simulink model "SID"  (R2017b)
settings: Solver=FixedStepAuto  StartTime=0.0  StopTime=inf  RelTol=1e-3  EnableMultiTasking=on
values from neighbouring files (symbols this model uses):
  Ad = Ad+Anew^i*Ts^i/factorial(i)    [SiD_Skript.m]
  Bd = pinv(Anew)*(Ad-eye(13))*Bnew    [SiD_Skript.m]
  Cd = C    [SiD_Skript.m]
  Dd = 0    [SiD_Skript.m]
  l = 0.175    [SiD_Skript.m]
libraries: WebSocketLibrary x1
settings Model: SimulationMode=external  Creator=seel  LastModifiedBy=jan
settings OptimizationCC: DefaultParameterBehavior=Inlined
settings DebuggingCC: MultiTaskCondExecSysMsg=warning  ParameterTunabilityLossMsg=error
settings SFSimCC: MATLABDynamicMemAlloc=off
settings RTWCC: SystemTargetFile=ert_linux.tlc  MakeCommand=make_rtw OPTS=-DWITH_HW  TemplateMakefile=ert_linux.tmf  Description=Linux Embedded Coder  GenerateReport=on  IncludeHyperlinkInReport=on  LaunchReport=on  TargetLang=C++  GenerateTraceInfo=on  GenerateTraceReport=on  GenerateTraceReportSl=on  GenerateTraceReportSf=on  GenerateTraceReportEml=on
settings CodeAppCC: ForceParamTrailComments=on  IgnoreCustomStorageClasses=off  OperatorAnnotations=on  SimulinkDataObjDesc=on  SFDataObjDesc=on  MATLABFcnDesc=on  InsertBlockDesc=on  StateflowObjectComments=on  MATLABSourceComments=on
settings STFCustomTargetCC: TargetLangStandard=C++03 (ISO)  ModelReferenceCompliant=off  CombineOutputUpdateFcns=on  ERTCustomFileBanners=on  SupportNonInlinedSFcns=off  RemoveResetFunc=on  SupportVariableSizeSignals=on  MATLABClassNameForMDSCustomization=Simulink.SoftwareTarget.ERTCustomization  GRTInterface=off  SystemTargetFile=ert_linux.tlc
settings ERTTargetCC: TargetLangStandard=C++03 (ISO)  MultiwordLength=2048  ModelReferenceCompliant=off  ParMdlRefBuildCompliant=off  CompOptLevelCompliant=off  ConcurrentExecutionCompliant=off  SupportContinuousTime=on  SupportVariableSizeSignals=on  ModelStepFunctionPrototypeControlCompliant=off  CPPClassGenCompliant=off  UseToolchainInfoCompliant=off  ExtMode=on  InlinedParameterPlacement=NonHierarchical  ERTCustomFileTemplate=ert_linux_file_process.tlc

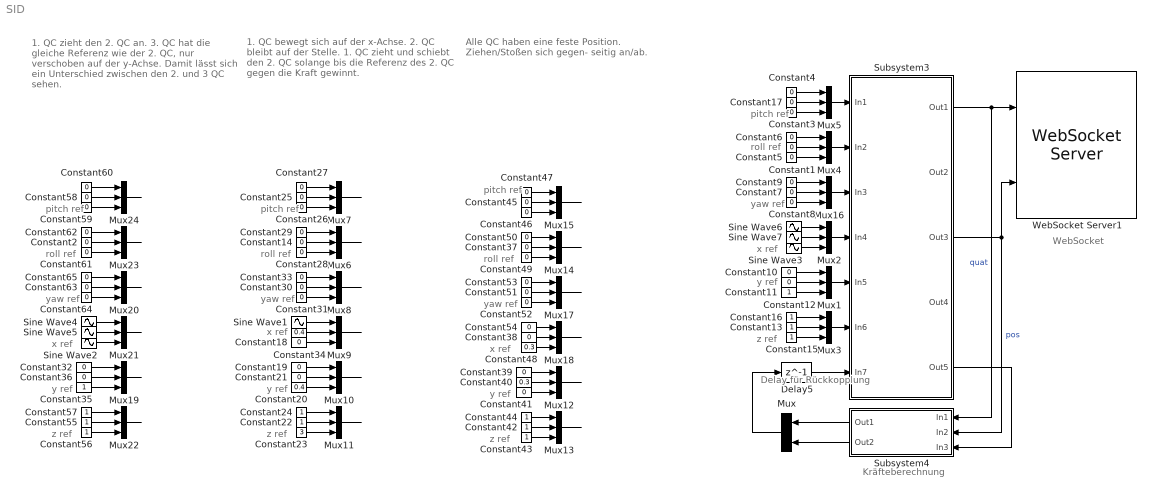
== system SID ==
  note: 1. QC bewegt sich auf der
      | x-Achse.
      | 2. QC bleibt auf der Stelle.
      | 1. QC zieht und schiebt den
      | 2. QC solange bis die Referenz
      | des 2. QC gegen die Kraft
      | gewinnt.
  note: WebSocket
  note: Delay für Rückkopplung
  note: Kräfteberechnung
  note: pitch ref
  note: x ref
  note: yaw ref
  note: roll ref
  note: z ref
  note: y ref
  note: pitch ref
  note: roll ref
  note: yaw ref
  note: z ref
  note: y ref
  note: x ref
  note: Alle QC haben eine feste Position.
      | Ziehen/Stoßen sich gegen-
      | seitig an/ab.
  note: 1. QC zieht den 2. QC an.
      | 3. QC hat die gleiche Referenz
      | wie der 2. QC, nur verschoben
      | auf der y-Achse.
      | Damit lässt sich ein Unterschied
      | zwischen den 2. und 3 QC sehen.
  note: z ref
  note: yaw ref
  note: roll ref
  note: y ref
  note: x ref
  note: pitch ref
  note: z ref
  note: yaw ref
  note: roll ref
  note: y ref
  note: x ref
  note: pitch ref
  Constant{1..10,12,14,17..19,21,25..33,36..39,41,45..47,49..54,58..65} (47 alike) : Constant  Value=0
  Constant{11,13,15..16,22,24,35,42..44,55..57} (13 alike) : Constant
  Constant20 : Constant  Value=0.4
  Constant23 : Constant  Value=3
  Constant34 : Constant  Value=0.4
  Constant40 : Constant  Value=0.3
  Constant48 : Constant  Value=0.3
  Delay5 : Delay  DelayLength=1  SampleTime=0.04
  Mux : Mux  Inputs=2
  Mux{1..24} (24 alike) : Mux  Inputs=3
  Sine Wave{1..3,5,7} (5 alike) : Sin  Bias=-0.15  Frequency=pi/15  SampleTime=0.04
  Sine Wave4 : Sin  Bias=-0.15  Frequency=pi/15  Phase=0.6  SampleTime=0.04
  Sine Wave6 : Sin  Bias=-0.15  Frequency=pi/15  Phase=0.6  SampleTime=0.04
  Subsystem3 : Subsystem
  Subsystem4 : Subsystem
  WebSocket Server1 : WebSocketLibrary/WebSocket Server  nOutputs=[1]  nInputs=[12,9]  splitInputs=[0,0]  jsonBlockConfig=''  totalSizeOut=7  totalSizeIn=7  nDiffInputs=6  address=localhost  port=30000  resource=/ws  sampleTime=0.04
  wires:
  Subsystem3/3(Out3) -> WebSocket Server1/2, Subsystem4/2(In2)  "pos"
  Mux/1 -> Delay5/1
  Subsystem3/1(Out1) -> WebSocket Server1/1, Subsystem4/1(In1)  "quat"
  Subsystem4/1(Out1) -> Mux/1
  Subsystem4/2(Out2) -> Mux/2
  Subsystem3/5(Out5) -> Subsystem4/3(In3)
  Delay5/1 -> Subsystem3/7(In7)
  Mux7/1 -> ?
  Constant18/1 -> Mux9/3
  Constant19/1 -> Mux10/1
  Sine Wave1/1 -> Mux9/1
  Constant24/1 -> Mux11/1
  Constant25/1 -> Mux7/2
  Constant23/1 -> Mux11/3
  Constant28/1 -> Mux6/3
  Mux11/1 -> ?
  Constant21/1 -> Mux10/2
  Constant33/1 -> Mux8/1
  Constant27/1 -> Mux7/1
  Constant29/1 -> Mux6/1
  Mux6/1 -> ?
  Constant30/1 -> Mux8/2
  Mux10/1 -> ?
  Constant20/1 -> Mux10/3
  Constant14/1 -> Mux6/2
  Constant31/1 -> Mux8/3
  Constant34/1 -> Mux9/2
  Mux9/1 -> ?
  Constant22/1 -> Mux11/2
  Mux8/1 -> ?
  Constant26/1 -> Mux7/3
  Constant40/1 -> Mux12/2
  Constant45/1 -> Mux15/2
  Mux12/1 -> ?
  Constant41/1 -> Mux12/3
  Constant47/1 -> Mux15/1
  Mux14/1 -> ?
  Mux15/1 -> ?
  Constant49/1 -> Mux14/3
  Constant53/1 -> Mux17/1
  Mux17/1 -> ?
  Constant38/1 -> Mux18/2
  Constant54/1 -> Mux18/1
  Constant52/1 -> Mux17/3
  Mux18/1 -> ?
  Constant44/1 -> Mux13/1
  Constant50/1 -> Mux14/1
  Constant43/1 -> Mux13/3
  Constant39/1 -> Mux12/1
  Constant46/1 -> Mux15/3
  Constant51/1 -> Mux17/2
  Constant37/1 -> Mux14/2
  Mux13/1 -> ?
  Constant48/1 -> Mux18/3
  Constant42/1 -> Mux13/2
  Constant12/1 -> Mux1/2
  Constant9/1 -> Mux16/1
  Constant5/1 -> Mux4/3
  Sine Wave7/1 -> Mux2/2
  Sine Wave6/1 -> Mux2/1
  Mux2/1 -> Subsystem3/4(In4)
  Constant4/1 -> Mux5/1
  Constant13/1 -> Mux3/2
  Constant10/1 -> Mux1/1
  Constant11/1 -> Mux1/3
  Constant8/1 -> Mux16/3
  Constant7/1 -> Mux16/2
  Sine Wave3/1 -> Mux2/3
  Mux4/1 -> Subsystem3/2(In2)
  Constant15/1 -> Mux3/3
  Constant17/1 -> Mux5/2
  Constant6/1 -> Mux4/1
  Mux16/1 -> Subsystem3/3(In3)
  Constant1/1 -> Mux4/2
  Constant16/1 -> Mux3/1
  Constant3/1 -> Mux5/3
  Mux1/1 -> Subsystem3/5(In5)
  Mux3/1 -> Subsystem3/6(In6)
  Mux5/1 -> Subsystem3/1(In1)
  Mux23/1 -> ?
  Constant59/1 -> Mux24/3
  Constant63/1 -> Mux20/2
  Mux20/1 -> ?
  Constant56/1 -> Mux22/3
  Sine Wave2/1 -> Mux21/3
  Constant60/1 -> Mux24/1
  Constant35/1 -> Mux19/3
  Constant36/1 -> Mux19/2
  Mux21/1 -> ?
  Constant65/1 -> Mux20/1
  Constant61/1 -> Mux23/3
  Mux19/1 -> ?
  Sine Wave4/1 -> Mux21/1
  Constant62/1 -> Mux23/1
  Constant32/1 -> Mux19/1
  Sine Wave5/1 -> Mux21/2
  Constant58/1 -> Mux24/2
  Constant64/1 -> Mux20/3
  Mux22/1 -> ?
  Constant57/1 -> Mux22/1
  Constant2/1 -> Mux23/2
  Mux24/1 -> ?
  Constant55/1 -> Mux22/2

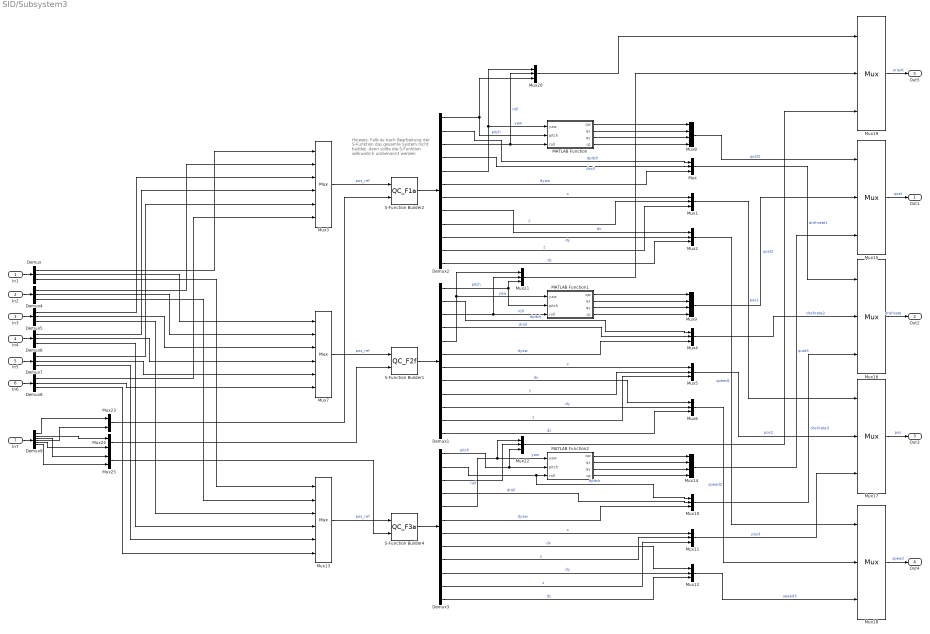
== system SID/Subsystem3 ==
  note: Hinweis: Falls es nach Bearbeitung der
      | S-Funktion das gesamte System
      | nicht buildet, dann sollte die S-Funktion
      | willkuerlich umbenannt werden
  In1 : Inport
  In2 : Inport  Port=2
  In3 : Inport  Port=3
  In4 : Inport  Port=4
  In5 : Inport  Port=5
  In6 : Inport  Port=6
  In7 : Inport  Port=7
  Demux{,4..8} (6 alike) : Demux  Outputs=3
  Demux1 : Demux  Outputs=12
  Demux2 : Demux  Outputs=12
  Demux3 : Demux  Outputs=12
  Demux9 : Demux  Outputs=6
  MATLAB Function : MATLAB Function  TreatAsAtomicUnit=on
  MATLAB Function1 : MATLAB Function  TreatAsAtomicUnit=on
  MATLAB Function2 : MATLAB Function  TreatAsAtomicUnit=on
  Mux{,1..2,4..6,10..12,15..22} (17 alike) : Mux  Inputs=3
  Mux13 : Mux  Inputs=6
  Mux14 : Mux
  Mux23 : Mux  Inputs=2
  Mux24 : Mux  Inputs=2
  Mux25 : Mux  Inputs=2
  Mux3 : Mux  Inputs=6
  Mux7 : Mux  Inputs=6
  Mux8 : Mux
  Mux9 : Mux
  S-Function Builder1 : S-Function  InitFcn=try, set_param(gcb,'FunctionName','QC_F2f'), end  FunctionName=QC_F2f  Parameters=Ad,Bd,Cd,Dd  SFunctionModules=QC_F2f_wrapper  SFunctionDeploymentMode=off  EnableBusSupport=off  mask(S-Function Builder){}
      mask help: Simulink:masks:SFunctionBuilder_MD
      mask init:
      | val = [[.9  0.75 0.75 1 1 .9 .9 1]',[1 1 0.75 0.75 .9 .9 1 .9]'];try , sys = get_param(gcb,'SfunBuilderFcnName');if isempty(sys), sys = get_param(gcb,'FunctionName'); end,catch, sys = get_param(gcb,'FunctionName'); end
      settings: CopyFcn=set_param(gcbh,'LinkStatus','none')  PreSaveFcn=try, set_param(gcb,'FunctionName','QC_F2f'), end  OpenFcn=sfunctionwizard(gcbh)
      mask Display: plot(val(:,1),val(:,2)),disp(sys), port_label('input',1,'u'), port_label('input',2,'F'), port_label('output',1,'y')
  S-Function Builder2 : S-Function  InitFcn=try, set_param(gcb,'FunctionName','QC_F1a'), end  FunctionName=QC_F1a  Parameters=Ad,Bd,Cd,Dd  SFunctionModules=QC_F1a_wrapper  SFunctionDeploymentMode=off  EnableBusSupport=off  mask(S-Function Builder){}
      mask help: Simulink:masks:SFunctionBuilder_MD
      mask init: same as SID/Subsystem3/S-Function Builder1
      settings: CopyFcn=set_param(gcbh,'LinkStatus','none')  PreSaveFcn=try, set_param(gcb,'FunctionName','QC_F1a'), end  OpenFcn=sfunctionwizard(gcbh)
      mask Display: plot(val(:,1),val(:,2)),disp(sys), port_label('input',1,'u'), port_label('input',2,'F'), port_label('output',1,'y')
  S-Function Builder4 : S-Function  InitFcn=try, set_param(gcb,'FunctionName','QC_F3a'), end  FunctionName=QC_F3a  Parameters=Ad,Bd,Cd,Dd  SFunctionModules=QC_F3a_wrapper  SFunctionDeploymentMode=off  EnableBusSupport=off  mask(S-Function Builder){}
      mask help: Simulink:masks:SFunctionBuilder_MD
      mask init: same as SID/Subsystem3/S-Function Builder1
      settings: CopyFcn=set_param(gcbh,'LinkStatus','none')  PreSaveFcn=try, set_param(gcb,'FunctionName','QC_F3a'), end  OpenFcn=sfunctionwizard(gcbh)
      mask Display: plot(val(:,1),val(:,2)),disp(sys), port_label('input',1,'u'), port_label('input',2,'F'), port_label('output',1,'y')
  Out1 : Outport
  Out2 : Outport  Port=2
  Out3 : Outport  Port=3
  Out4 : Outport  Port=4
  Out5 : Outport  Port=5
  wires:
  MATLAB Function/4(qz) -> Mux8/4
  MATLAB Function/3(qy) -> Mux8/3
  MATLAB Function/2(qx) -> Mux8/2
  MATLAB Function/1(qw) -> Mux8/1
  In1/1 -> Demux/1
  Mux3/1 -> S-Function Builder2/1  "pos_ref"
  S-Function Builder2/1 -> Demux2/1
  Demux2/1 -> Mux20/3, MATLAB Function/2(pitch)  "pitch"
  Demux2/3 -> MATLAB Function/3(roll), Mux20/2  "roll"
  Demux2/5 -> Mux20/1, MATLAB Function/1(yaw)  "yaw"
  Demux2/2 -> Mux/1  "dpitch"
  Demux2/4 -> Mux/2  "droll"
  Demux2/6 -> Mux/3  "dyaw"
  Demux2/7 -> Mux1/1  "x"
  Demux2/9 -> Mux1/2  "y"
  Demux2/11 -> Mux1/3  "z"
  Demux2/8 -> Mux2/1  "dx"
  Demux2/10 -> Mux2/2  "dy"
  Demux2/12 -> Mux2/3  "dz"
  Demux/1 -> Mux3/1
  Demux1/9 -> Mux5/2  "y"
  Demux1/10 -> Mux6/2  "dy"
  MATLAB Function1/4(qz) -> Mux9/4
  MATLAB Function1/3(qy) -> Mux9/3
  Demux1/11 -> Mux5/3  "z"
  MATLAB Function1/1(qw) -> Mux9/1
  Demux1/2 -> Mux4/1  "dpitch"
  Mux7/1 -> S-Function Builder1/1  "pos_ref"
  Demux1/1 -> MATLAB Function1/2(pitch), Mux21/3  "pitch"
  Demux1/12 -> Mux6/3  "dz"
  Demux1/7 -> Mux5/1  "x"
  Demux1/8 -> Mux6/1  "dx"
  Demux1/4 -> Mux4/2  "droll"
  MATLAB Function1/2(qx) -> Mux9/2
  Demux1/6 -> Mux4/3  "dyaw"
  Demux1/5 -> Mux21/1, MATLAB Function1/1(yaw)  "yaw"
  Demux1/3 -> Mux21/2, MATLAB Function1/3(roll)  "roll"
  Demux/2 -> Mux7/1
  Demux3/9 -> Mux11/2  "y"
  Demux3/10 -> Mux12/2  "dy"
  MATLAB Function2/4(qz) -> Mux14/4
  MATLAB Function2/3(qy) -> Mux14/3
  Demux3/11 -> Mux11/3  "z"
  MATLAB Function2/1(qw) -> Mux14/1
  Demux3/2 -> Mux10/1, MATLAB Function2/3(roll)  "dpitch"
  Mux13/1 -> S-Function Builder4/1  "pos_ref"
  Demux3/1 -> MATLAB Function2/2(pitch), Mux22/3  "pitch"
  Demux3/12 -> Mux12/3  "dz"
  Demux3/7 -> Mux11/1  "x"
  Demux3/8 -> Mux12/1  "dx"
  Demux3/4 -> Mux10/2  "droll"
  MATLAB Function2/2(qx) -> Mux14/2
  Demux3/6 -> Mux10/3  "dyaw"
  Demux3/5 -> MATLAB Function2/1(yaw), Mux22/1  "yaw"
  Demux3/3 -> Mux22/2  "roll"
  Demux/3 -> Mux13/1
  In2/1 -> Demux4/1
  In3/1 -> Demux5/1
  In4/1 -> Demux6/1
  In5/1 -> Demux7/1
  In6/1 -> Demux8/1
  Demux4/1 -> Mux3/2
  Demux4/2 -> Mux7/2
  Demux4/3 -> Mux13/2
  Demux5/1 -> Mux3/3
  Demux5/2 -> Mux7/3
  Demux5/3 -> Mux13/3
  Demux6/1 -> Mux3/4
  Demux7/1 -> Mux3/5
  Demux8/1 -> Mux3/6
  Demux6/2 -> Mux7/4
  Demux7/2 -> Mux7/5
  Demux8/2 -> Mux7/6
  Demux6/3 -> Mux13/4
  Demux7/3 -> Mux13/5
  Demux8/3 -> Mux13/6
  Mux8/1 -> Mux15/1  "quat1"
  Mux9/1 -> Mux15/2  "quat2"
  Mux14/1 -> Mux15/3  "quat3"
  Mux/1 -> Mux16/1  "drehrate1"
  Mux4/1 -> Mux16/2  "drehrate2"
  Mux10/1 -> Mux16/3  "drehrate3"
  Mux1/1 -> Mux17/1  "pos1"
  Mux5/1 -> Mux17/2  "pos2"
  Mux11/1 -> Mux17/3  "pos3"
  Mux2/1 -> Mux18/1  "speed1"
  Mux6/1 -> Mux18/2  "speed2"
  Mux12/1 -> Mux18/3  "speed3"
  Mux15/1 -> Out1/1  "quat"
  Mux16/1 -> Out2/1  "drehrate"
  Mux17/1 -> Out3/1  "pos"
  Mux18/1 -> Out4/1  "speed"
  Mux20/1 -> Mux19/1
  Mux21/1 -> Mux19/2
  Mux22/1 -> Mux19/3
  Mux19/1 -> Out5/1  "orient"
  In7/1 -> Demux9/1
  S-Function Builder1/1 -> Demux1/1
  S-Function Builder4/1 -> Demux3/1
  Demux9/1 -> Mux23/1
  Demux9/2 -> Mux24/1
  Demux9/3 -> Mux25/1
  Demux9/4 -> Mux23/2
  Demux9/5 -> Mux24/2
  Demux9/6 -> Mux25/2
  Mux23/1 -> S-Function Builder2/2
  Mux24/1 -> S-Function Builder1/2
  Mux25/1 -> S-Function Builder4/2

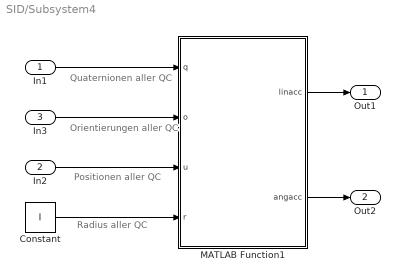
== system SID/Subsystem4 ==
  note: Positionen aller QC
  note: Radius aller QC
  note: Orientierungen aller QC
  note: Quaternionen aller QC
  In1 : Inport
  In2 : Inport  Port=2
  In3 : Inport  Port=3
  Constant : Constant  Value=l  SampleTime=0.04
  MATLAB Function1 : MATLAB Function  TreatAsAtomicUnit=on
  Out1 : Outport
  Out2 : Outport  Port=2
  wires:
  Constant/1 -> MATLAB Function1/4(r)
  MATLAB Function1/1(linacc) -> Out1/1
  In1/1 -> MATLAB Function1/1(q)
  In2/1 -> MATLAB Function1/3(u)
  In3/1 -> MATLAB Function1/2(o)
  MATLAB Function1/2(angacc) -> Out2/1

== matlab function SID/Subsystem4/MATLAB Function1 ==
  data: q input; o input; u input; linacc output; r input; angacc output
% Projekt: SiD
% Autoren: Jan-Philip Wirsching, Aarohan Jain
% Betreuer: Dr. Ing Thomas Seel, Karsten Eckhoff
% Sommersemester 2019
% 05.08.2019

% MATLAB-Funktion zur Berechnung von
% abstossenden und anziehenden Kraeften
% zwischen 2 Quadrocoptern.
% linacc ist die gesamte Kraft, die
% die x,y,z Positionen betrifft
% angacc ist die gesamte Kraft, die
% die pitch,roll,yaw Orientierungen
% betrifft.

function [linacc, angacc] = fcn(q,o,u,r) % Eingang: quat, orientierung, pos, radius
    n=3; % Anzahl von QC (Zaehler fuer Index i)
    N=3; % Zaehler fuer Index j
    
    kraft=zeros(9,1); % Init aller gebrauchten Kraft-Vektoren
    krafttemp=zeros(n,1);
    kraftanz = zeros(n,1);
    kraftanz2 = zeros(n,1);
    angacctemp = zeros(9,1);
    angacc = zeros(9,1);
    
    k = 0.05; % Skalierung der anziehenden Kraft
    k2 = 1; % Skalierung der abstossenden Kraft
    
    di = [r;0;0]'; % Position vom 1. Magneten (lokal)
    dj = [r;0;0]';
    di2 = [-r;0;0]'; % Position vom 2. Magneten (lokal)
    dj2 = [-r;0;0]';
    
    for i=1:n
        quati = q(4*i-3:4*i)';
        for j=1:N
            if (i ~= j)                    
                quatj = q(4*j-3:4*j)';
                dgi = ((u(3*i-2:3*i))' + quaternionRotate(quati,di))'; % Umwandlung in globale Koordinaten (Mag1)
                dgj = ((u(3*j-2:3*j))' + quaternionRotate(quatj,dj))'; 
                
                % ANZIEHUNG
               % if (norm(u((3*i-2):3*i)-u((3*j-2):3*j))<=3*r) % Anziehungskraft wirkt wenn Abstand zw 2 QC kleiner als 3*radius               
               if(norm(dgi-dgj)<=3*r) % Anziehungskraft wirkt wenn Abstand zw 2 Magneten kleiner als 3*radius
                    dgi2 = ((u(3*i-2:3*i))' + quaternionRotate(quati,di2))'; % Umwandlung in globale Koordinaten (Mag2)
                    dgj2 = ((u(3*j-2:3*j))' + quaternionRotate(quatj,dj2))';
                    kraftanz = k*((dgj-dgi)/(norm(dgj-dgi))) * 1*((norm(dgj-dgi))^2); % Anz. Kraft vom 1. Magneten
                    kraftanz2 = k*((dgj2-dgi2)/(norm(dgj2-dgi2))) * 1*((norm(dgj2-dgi2))^2); % Anz. Kraft vom 2. Magneten
                    kraft(3*i-2:3*i) = kraft((3*i-2):3*i) + kraftanz + kraftanz2; % Kraft = Fruehere Kraft + neue Kraft
               end
                
               
                % ABSTOSSUNG
                if (norm(u((3*i-2):3*i)-u((3*j-2):3*j))<=2*r) % Abstossende Kraft wirkt wenn Abstand zw 2 QC kleiner als 2*radius
                    tiefe = 2*r-norm(u((3*i-2):3*i)-u((3*j-2):3*j)); % Eindringtiefe 
                    richtung = (u((3*i-2):3*i)-u((3*j-2):3*j))/norm(u((3*i-2):3*i)-u((3*j-2):3*j));
                    krafttemp = k2*tiefe*tiefe*richtung; % Willkuerlich gewaehlte Beziehung zw Kraft und Eindringtiefe
                    kraft(3*i-2:3*i) = kraft((3*i-2):3*i) + krafttemp; % Kraft = Fruehere Kraft + neue Kraft
                end
            
            end
        end
        angacctemp(3*i-2:3*i) = cross(quaternionRotate(quati,di),kraft(3*i-2:3*i)); % Winkelbeschleunigung/Kraft
        
        rotmat = [1 tand(o(3*i-1))*sind(o(3*i-2)) cosd(o(3*i-2))*tand(o(3*i-1)); 0 cosd(o(3*i-1)) -sind(o(3*i-1)); 0 sind(o(3*i-1))*cosd(o(3*i-2)) cosd(o(3*i-1))*cosd(o(3*i-2))];
        % Quelle: https://davidbrown3.github.io/2017-07-25/EulerAngles/
        % (Zugriff: 05.08.2019)
        
        angacc(3*i-2:3*i) = 1*rotmat*angacctemp(3*i-2:3*i);
    end
    linacc = 1*kraft;
end

== matlab function SID/Subsystem3/MATLAB Function ==
  data: yaw input; qw output; pitch input; roll input; qx output; qy output; qz output
% Projekt: SiD
% Autoren: Jan-Philip Wirsching, Aarohan Jain
% Betreuer: Dr. Ing Thomas Seel, Karsten Eckhoff
% Sommersemester 2019
% 05.08.2019

% MATLAB-Funktion zur Umrechnung von 
% Euler Winkeln (roll, pitch, yaw) zu
% Quaternionen (qw, qz, qy, qx)

function [qw,qx,qy,qz] = fcn(yaw, pitch, roll)
    cy = cosd(yaw*0.5);
    sy = sind(yaw*0.5);
    cp = cosd(pitch*0.5);
    sp = sind(pitch*0.5);
    cr = cosd(roll*0.5);
    sr = sind(roll*0.5);
    
    qw = cy*cp*cr + sy*sp*sr;
    qz = cy*cp*sr - sy*sp*cr;
    qy = (sy*cp*sr + cy*sp*cr);
    qx = (sy*cp*cr - cy*sp*sr);
end

== matlab function SID/Subsystem3/MATLAB Function1 ==
  data: yaw input; qw output; pitch input; roll input; qx output; qy output; qz output
% Projekt: SiD
% Autoren: Jan-Philip Wirsching, Aarohan Jain
% Betreuer: Dr. Ing Thomas Seel, Karsten Eckhoff
% Sommersemester 2019
% 05.08.2019

% MATLAB-Funktion zur Umrechnung von 
% Euler Winkeln (roll, pitch, yaw) zu
% Quaternionen (qw, qz, qy, qx)

function [qw,qx,qy,qz] = fcn(yaw, pitch, roll)
    cy = cosd(yaw*0.5);
    sy = sind(yaw*0.5);
    cp = cosd(pitch*0.5);
    sp = sind(pitch*0.5);
    cr = cosd(roll*0.5);
    sr = sind(roll*0.5);
    
    qw = cy*cp*cr + sy*sp*sr;
    qz = cy*cp*sr - sy*sp*cr;
    qy = (sy*cp*sr + cy*sp*cr);
    qx = (sy*cp*cr - cy*sp*sr);
end

== matlab function SID/Subsystem3/MATLAB Function2 ==
  data: yaw input; qw output; pitch input; roll input; qx output; qy output; qz output
% Projekt: SiD
% Autoren: Jan-Philip Wirsching, Aarohan Jain
% Betreuer: Dr. Ing Thomas Seel, Karsten Eckhoff
% Sommersemester 2019
% 05.08.2019

% MATLAB-Funktion zur Umrechnung von 
% Euler Winkeln (roll, pitch, yaw) zu
% Quaternionen (qw, qz, qy, qx)

function [qw,qx,qy,qz] = fcn(yaw, pitch, roll)
    cy = cosd(yaw*0.5);
    sy = sind(yaw*0.5);
    cp = cosd(pitch*0.5);
    sp = sind(pitch*0.5);
    cr = cosd(roll*0.5);
    sr = sind(roll*0.5);
    
    qw = cy*cp*cr + sy*sp*sr;
    qz = cy*cp*sr - sy*sp*cr;
    qy = (sy*cp*sr + cy*sp*cr);
    qx = (sy*cp*cr - cy*sp*sr);
end
